simulink model "InductionCookerStateFlow_HarnessButtonS1"  (R2023a)
settings: Solver=FixedStepDiscrete  StartTime=0.0  StopTime=200  FixedStep=0.1  RelTol=1e-3  EnableMultiTasking=on
settings Model: Creator=anton  LastModifiedBy=anton
settings SolverCC: AlgebraicLoopSolver=TrustRegion  AutoInsertRateTranBlk=on
settings DataIOCC: LimitDataPoints=on
settings OptimizationCC: LifeSpan=inf
settings DebuggingCC: UnconnectedInputMsg=warning  UnconnectedOutputMsg=warning  UnconnectedLineMsg=warning  AllowSymbolicDim=off  SFUnexpectedBacktrackingDiag=warning  SFNoUnconditionalDefaultTransitionDiag=warning  SFExecutionAtInitializationDiag=none  ArithmeticOperatorsInVariantConditions=warning
settings ModelReferenceCC: EnableRefExpFcnMdlSchedulingChecks=on
settings SFSimCC: SimUseLocalCustomCode=off  CustomCodeUndefinedFunction=UseInterfaceOnly
settings RTWCC: RTWUseLocalCustomCode=off  DLArmComputeVersion=19.05
settings CodeAppCC: StateflowObjectComments=on
settings GRTTargetCC: TargetLangStandard=C89/C90 (ANSI)
settings ConfigComp: CovEnable=on  RecordCoverage=on  CovMetricSettings=dw  CovSaveCumulativeToWorkspaceVar=on  CovSaveSingleToWorkspaceVar=on  CovModelRefEnable=on

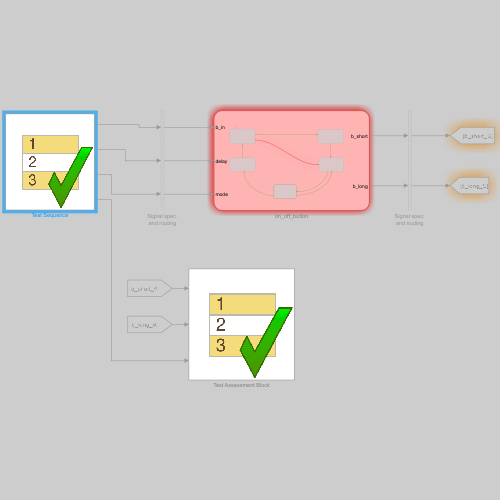
[thumbnail: Simulink's stored preview of the top-level diagram]
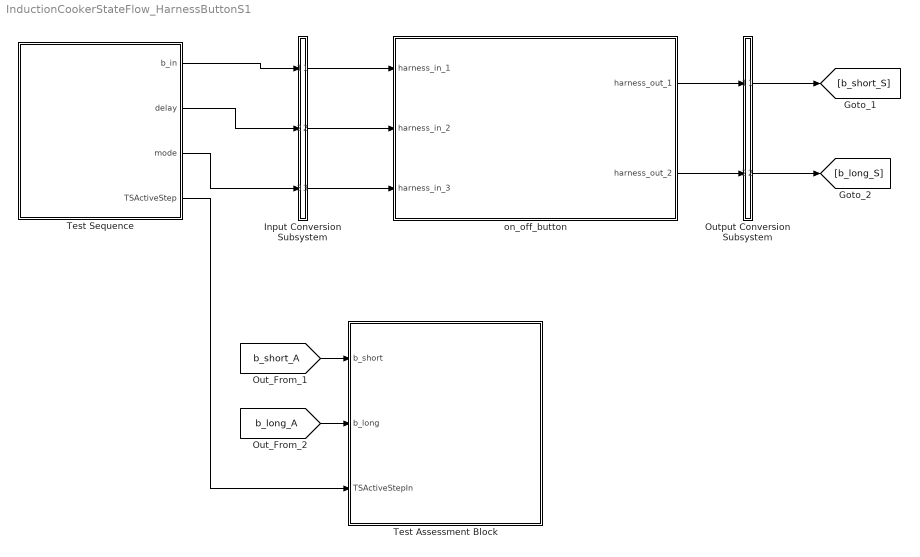
== system InductionCookerStateFlow_HarnessButtonS1 ==
  Input Conversion Subsystem : Subsystem  Tag=__SLT_ICS__  Description=|
      | Signal spec.
      | and routing
      settings: AttributesFormatString=%<Description>
  Output Conversion Subsystem : Subsystem  Tag=__SLT_OCS__  Description=|
      | Signal spec.
      | and routing
      settings: AttributesFormatString=%<Description>
  Test Assessment Block : Test Sequence  Tag=__SLT_ASMT__  TreatAsAtomicUnit=on
  Test Sequence : Test Sequence  TreatAsAtomicUnit=on
  on_off_button : Subsystem  Tag=__SL_testing_harness_stub_
  wires:
  [b_short_A] -> Test Assessment Block/1(b_short)
  [b_long_A] -> Test Assessment Block/2(b_long)
  Test Sequence/1(b_in) -> Input Conversion Subsystem/1(Inport_1)
  Test Sequence/2(delay) -> Input Conversion Subsystem/2(Inport_2)
  Test Sequence/3(mode) -> Input Conversion Subsystem/3(Inport_3)
  Output Conversion Subsystem/1(Outport_1) -> [b_short_S]
  Output Conversion Subsystem/2(Outport_2) -> [b_long_S]
  Test Sequence/4(TSActiveStep) -> Test Assessment Block/3(TSActiveStepIn)
  on_off_button/1(harness_out_1) -> Output Conversion Subsystem/1(Inport_1)
  on_off_button/2(harness_out_2) -> Output Conversion Subsystem/2(Inport_2)
  Input Conversion Subsystem/1(Outport_1) -> on_off_button/1(harness_in_1)
  Input Conversion Subsystem/2(Outport_2) -> on_off_button/2(harness_in_2)
  Input Conversion Subsystem/3(Outport_3) -> on_off_button/3(harness_in_3)

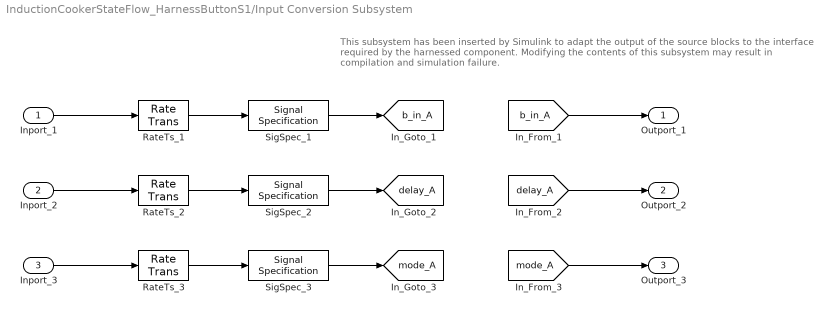
== system InductionCookerStateFlow_HarnessButtonS1/Input Conversion Subsystem ==
  note: This subsystem has been inserted by Simulink to adapt the output of the source blocks to the interface required by the harnessed component.
      |  Modifying the contents of this subsystem may result in compilation and simulation failure.
  Inport_1 : Inport
  Inport_2 : Inport  Port=2
  Inport_3 : Inport  Port=3
  RateTs_1 : RateTransition  OutPortSampleTime=0.1
  RateTs_2 : RateTransition  OutPortSampleTime=[-1, 0]
  RateTs_3 : RateTransition  OutPortSampleTime=[-1, 0]
  SigSpec_1 : SignalSpecification  OutDataTypeStr=boolean  Dimensions=[1]  SampleTime=0.1
  SigSpec_2 : SignalSpecification  OutDataTypeStr=double  Dimensions=[1]  SampleTime=[-1, 0]
  SigSpec_3 : SignalSpecification  OutDataTypeStr=uint8  Dimensions=[1]  SampleTime=[-1, 0]
  Outport_1 : Outport
  Outport_2 : Outport  Port=2
  Outport_3 : Outport  Port=3
  tag scope: b_in_A=global, delay_A=global, mode_A=global
  wires:
  [b_in_A] -> Outport_1/1
  SigSpec_1/1 -> [b_in_A]
  RateTs_1/1 -> SigSpec_1/1
  Inport_1/1 -> RateTs_1/1
  [delay_A] -> Outport_2/1
  SigSpec_2/1 -> [delay_A]
  RateTs_2/1 -> SigSpec_2/1
  Inport_2/1 -> RateTs_2/1
  [mode_A] -> Outport_3/1
  SigSpec_3/1 -> [mode_A]
  RateTs_3/1 -> SigSpec_3/1
  Inport_3/1 -> RateTs_3/1

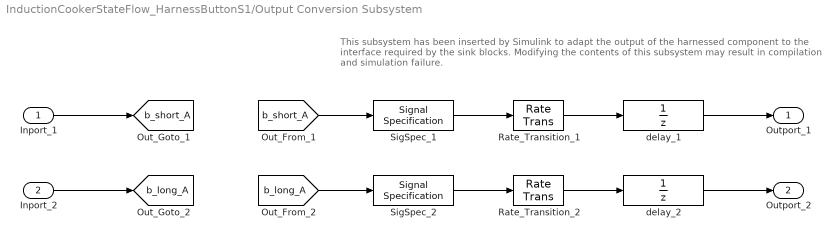
== system InductionCookerStateFlow_HarnessButtonS1/Output Conversion Subsystem ==
  note: This subsystem has been inserted by Simulink to adapt the output of the harnessed component to the interface required by the sink blocks.
      |  Modifying the contents of this subsystem may result in compilation and simulation failure.
  Inport_1 : Inport
  Inport_2 : Inport  Port=2
  Rate_Transition_1 : RateTransition  OutPortSampleTimeOpt=Inherit
  Rate_Transition_2 : RateTransition  OutPortSampleTimeOpt=Inherit
  SigSpec_1 : SignalSpecification  OutDataTypeStr=boolean  Dimensions=[1]  SampleTime=0.1
  SigSpec_2 : SignalSpecification  OutDataTypeStr=boolean  Dimensions=[1]  SampleTime=0.1
  delay_1 : UnitDelay  SampleTime=-1
  delay_2 : UnitDelay  SampleTime=-1
  Outport_1 : Outport
  Outport_2 : Outport  Port=2
  tag scope: b_long_A=global, b_short_A=global
  wires:
  Inport_1/1 -> [b_short_A]
  [b_short_A] -> SigSpec_1/1
  SigSpec_1/1 -> Rate_Transition_1/1
  Rate_Transition_1/1 -> delay_1/1
  delay_1/1 -> Outport_1/1
  Inport_2/1 -> [b_long_A]
  [b_long_A] -> SigSpec_2/1
  SigSpec_2/1 -> Rate_Transition_2/1
  Rate_Transition_2/1 -> delay_2/1
  delay_2/1 -> Outport_2/1

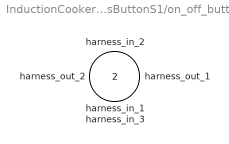
== system InductionCookerStateFlow_HarnessButtonS1/on_off_button ==
  harness_in_1 : Inport
  harness_in_2 : Inport  Port=2
  harness_in_3 : Inport  Port=3
  harness_out_1 : Outport
  harness_out_2 : Outport  Port=2

== stateflow chart InductionCookerStateFlow_HarnessButtonS1/Test Assessment Block ==
  state Scenario_1
    state Run
      state VerifyInit_S1
        verify(b_long & b_short);
      state VerifyButtonFirstPressed_S1
        verify(~b_short & b_long);
      state VerifyButtonFirstPressedWait_S1
        verify(~b_short & b_long);
      state VerifyButtonFirstReleased_S1
        verify(b_short & b_long);
      state VerifyButtonFirstReleasedWait_S1
        verify(b_short & b_long);
      state VerifyButtonShortPressed_S1
        verify(b_short & b_long);
      state VerifyButtonSecondReleased_S1
        verify(b_short & b_long);
      state VerifyButtonFirstLongPressed_S1
        state VerifyButtonFirstLongPressed_1_S1
          verify(b_short & b_long)
        state VerifyButtonFirstLongPressed_2_S1
          verify(b_short & ~b_long)
        (default) -> VerifyButtonFirstLongPressed_1_S1
        VerifyButtonFirstLongPressed_1_S1 -> VerifyButtonFirstLongPressed_2_S1 : [
            | after(1,sec)
            | ]
      state VerifyButtonSecondLongPressed_S1
        verify(b_short & b_long);
      state VerifyButtonSecondLongPressedWait_S1
        verify(b_short & b_long);
      state VerifyButtonThirdReleased_S1
        verify(b_short & b_long);
      state step_1_2
      (default) -> (junction 105)
      Run -> (junction 105)
      (junction 105) -> (junction 106) [order 1] : [TSActiveStepIn == TSActiveStepEnumButton.Init_S1
          | ]
      (junction 106) -> VerifyInit_S1 [order 1] : [~in(Scenario_1.Run.VerifyInit_S1)]
      (junction 105) -> (junction 114) [order 2]
      (junction 106) -> (junction 109) [order 2]
      (junction 114) -> (junction 115) [order 1] : [TSActiveStepIn == TSActiveStepEnumButton.ButtonFirstPressed_S1
          | ]
      (junction 115) -> VerifyButtonFirstPressed_S1 [order 1] : [~in(Scenario_1.Run.VerifyButtonFirstPressed_S1)]
      (junction 114) -> (junction 345) [order 2]
      (junction 115) -> (junction 118) [order 2]
      (junction 345) -> (junction 346) [order 1] : [TSActiveStepIn == TSActiveStepEnumButton.ButtonFirstPressedWait_S1
          | ]
      (junction 346) -> VerifyButtonFirstPressedWait_S1 [order 1] : [~in(Scenario_1.Run.VerifyButtonFirstPressedWait_S1)]
      (junction 345) -> (junction 122) [order 2]
      (junction 346) -> (junction 349) [order 2]
      (junction 122) -> (junction 123) [order 1] : [TSActiveStepIn == TSActiveStepEnumButton.ButtonFirstReleased_S1
          | ]
      (junction 123) -> VerifyButtonFirstReleased_S1 [order 1] : [~in(Scenario_1.Run.VerifyButtonFirstReleased_S1)]
      (junction 364) -> (junction 130) [order 2]
      (junction 123) -> (junction 126) [order 2]
      (junction 364) -> (junction 365) [order 1] : [TSActiveStepIn == TSActiveStepEnumButton.ButtonFirstReleasedWait_S1
          | ]
      (junction 365) -> VerifyButtonFirstReleasedWait_S1 [order 1] : [~in(Scenario_1.Run.VerifyButtonFirstReleasedWait_S1)]
      (junction 130) -> (junction 131) [order 1] : [TSActiveStepIn == TSActiveStepEnumButton.ButtonShortPressed_S1
          | ]
      (junction 131) -> VerifyButtonShortPressed_S1 [order 1] : [~in(Scenario_1.Run.VerifyButtonShortPressed_S1)]
      (junction 130) -> (junction 138) [order 2]
      (junction 131) -> (junction 134) [order 2]
      (junction 138) -> (junction 139) [order 1] : [TSActiveStepIn == TSActiveStepEnumButton.ButtonSecondReleased_S1
          | ]
      (junction 139) -> VerifyButtonSecondReleased_S1 [order 1] : [~in(Scenario_1.Run.VerifyButtonSecondReleased_S1)]
      (junction 138) -> (junction 147) [order 2]
      (junction 139) -> (junction 142) [order 2]
      (junction 147) -> (junction 148) [order 1] : [TSActiveStepIn == TSActiveStepEnumButton.ButtonFirstLongPressed_S1
          | ]
      (junction 148) -> VerifyButtonFirstLongPressed_S1 [order 1] : [~in(Scenario_1.Run.VerifyButtonFirstLongPressed_S1)]
      (junction 147) -> (junction 155) [order 2]
      (junction 148) -> (junction 151) [order 2]
      (junction 155) -> (junction 156) [order 1] : [TSActiveStepIn == TSActiveStepEnumButton.ButtonSecondLongPressed_S1
          | ]
      (junction 156) -> VerifyButtonSecondLongPressed_S1 [order 1] : [~in(Scenario_1.Run.VerifyButtonSecondLongPressed_S1)]
      (junction 155) -> (junction 354) [order 2]
      (junction 156) -> (junction 159) [order 2]
      (junction 354) -> (junction 355) [order 1] : [TSActiveStepIn == TSActiveStepEnumButton.ButtonSecondLongPressedWait_S1
          | ]
      (junction 355) -> VerifyButtonSecondLongPressedWait_S1 [order 1] : [~in(Scenario_1.Run.VerifyButtonSecondLongPressedWait_S1)]
      (junction 354) -> (junction 164) [order 2]
      (junction 355) -> (junction 358) [order 2]
      (junction 164) -> (junction 165) [order 1] : [TSActiveStepIn == TSActiveStepEnumButton.ButtonThirdReleased_S1
          | ]
      (junction 165) -> VerifyButtonThirdReleased_S1 [order 1] : [~in(Scenario_1.Run.VerifyButtonThirdReleased_S1)]
      (junction 164) -> (junction 174) [order 2]
      (junction 165) -> (junction 168) [order 2]
      (junction 174) -> (junction 175)
      (junction 175) -> step_1_2 [order 1] : [~in(Scenario_1.Run.step_1_2)]
      (junction 175) -> (junction 178) [order 2]
      (junction 365) -> (junction 368) [order 2]
      (junction 122) -> (junction 364) [order 2]
    (default) -> Run
  (default) -> Scenario_1 : {assert(Active_Scenario_Index == 1,'The value of Scenario Parameter ''Active_Scenario_Index'' is not valid. Use the index of the scenario to specify it.')}
  data: b_short input boolean size=[1]; b_long input boolean size=[1]; TSActiveStepIn input; Active_Scenario_Index parameter =1

== stateflow chart InductionCookerStateFlow_HarnessButtonS1/Test Sequence ==
  settings: updateMethod=DISCRETE  sampleTime=0.1
  state Scenario_1
    state Init_S1
      %% Initialize data outputs.
      b_in = true;
      delay = 1;
      mode = uint8(0);
      settings: description=|
          | Rappresenta la situazione iniziale in cui il pulsante non è
          | ancora premuto e la modalità operativa selezionata (0)
          | è quella di accensione/spegnimento.
    state ButtonFirstPressed_S1
      b_in = false;
      delay = 1;
      mode = uint8(0);
      settings: description=Pressione del pulsante.
    state ButtonFirstPressedWait_S1
      b_in = false;
      delay = 1;
      mode = uint8(0);
      settings: description=|
          | Pressione del pulsante per coprire il caso in cui la
          | transizione sia falsa.
    state ButtonFirstReleased_S1
      b_in = true;
      delay = 1;
      mode = uint8(0);
      settings: description=|
          | Situazione in cui, dopo la pressione, avviene il rilascio
          | del pulsante.
    state ButtonFirstReleasedWait_S1
      b_in = true;
      delay = 1;
      mode = uint8(0);
      settings: description=|
          | Rilascio del pulsante per coprire il caso in cui la
          | transizione sia falsa.
    state ButtonShortPressed_S1
      b_in = false;
      delay = 1;
      mode = uint8(0);
      settings: description=|
          | Dallo step precedente, in cui ho rilasciato il pulsante,
          | effettuo una nuova pressione considerando questo step
          | attivo per 0.5 secondi. Mi aspetto che il livello alto non
          | venga raggiunto.
    state ButtonSecondReleased_S1
      b_in = true;
      delay = 1;
      mode = uint8(0);
      settings: description=Rilascio del pulsante dallo step precedente.
    state ButtonFirstLongPressed_S1
      b_in = false;
      delay = 1;
      mode = uint8(0);
      settings: description=|
          | Pressione del pulsante per un secondo e mezzo.
          | Mi aspetto che il livello alto del pulsante venga raggiunto,
          | in quanto la pressione viene effettuata per almeno
          | 1 secondo.
    state ButtonSecondLongPressed_S1
      b_in = false;
      delay = 1;
      mode = uint8(0);
      settings: description=Catturo l'uscita b_long = PRESSED.
    state ButtonSecondLongPressedWait_S1
      b_in = false;
      delay = 1;
      mode = uint8(0);
      settings: description=|
          | Pressione del pulsante per coprire il caso in cui la
          | transizione sia falsa.
    state ButtonThirdReleased_S1
      b_in = true;
      delay = 1;
      mode = uint8(0);
      settings: description=Rilascio del pulsante.
    (default) -> Init_S1
    Init_S1 -> ButtonFirstPressed_S1 : [
        | true
        | ]
    ButtonFirstPressed_S1 -> ButtonFirstPressedWait_S1 : [
        | true
        | ]
    ButtonFirstPressedWait_S1 -> ButtonFirstReleased_S1 : [
        | true
        | ]
    ButtonFirstReleased_S1 -> ButtonFirstReleasedWait_S1 : [
        | true
        | ]
    ButtonFirstReleasedWait_S1 -> ButtonShortPressed_S1 : [
        | true
        | ]
    ButtonShortPressed_S1 -> ButtonSecondReleased_S1 : [
        | after(0.5, sec)
        | ]
    ButtonSecondReleased_S1 -> ButtonFirstLongPressed_S1 : [
        | true
        | ]
    ButtonFirstLongPressed_S1 -> ButtonSecondLongPressed_S1 : [
        | after(delay+sampleTime, sec)
        | ]
    ButtonSecondLongPressed_S1 -> ButtonSecondLongPressedWait_S1 : [
        | true
        | ]
    ButtonSecondLongPressedWait_S1 -> ButtonThirdReleased_S1 : [
        | true
        | ]
  (default) -> Scenario_1 : {assert(Active_Scenario_Index == 1,'The value of Scenario Parameter ''Active_Scenario_Index'' is not valid. Use the index of the scenario to specify it.')}
  data: b_in output boolean size=[1]; delay output double size=[1]; mode output uint8 size=[1]; TSActiveStep output Enum: TSActiveStepEnumButton; sampleTime constant double =str2num(get_param('InductionCoockerStateFlow','FixedStep')); Active_Scenario_Index parameter =1
